simulink model "recordEEGExpe3"  (R2019a)
settings: Solver=VariableStepAuto  StartTime=0.0  StopTime=1000  RelTol=1e-3
undefined symbols (not defined in the file or in its folder): daq
libraries: dsparch4 x3, daqlib x1, dspnetwork x1
settings Model: Creator=Kusunoki  LastModifiedBy=Owner

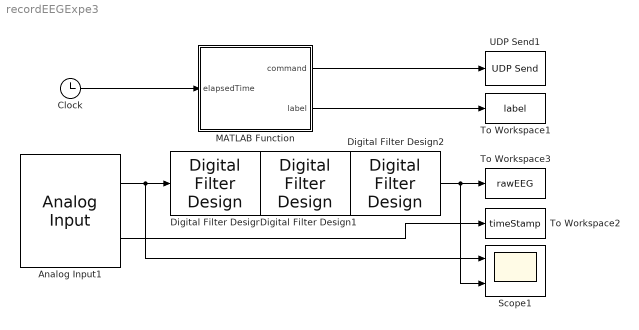
== system recordEEGExpe3 ==
  Analog Input1 : daqlib/Analog Input  DeviceMenu=ni Dev1 (USB-6000)  Device=ni Dev1 (USB-6000)  ObjConstructor=daq.createSession('ni')  NChannelsSelected=8  Channels=1$ai0$$Dev1$1$1$1$1$#1$ai1$$Dev1$1$1$1$1$#1$ai2$$Dev1$1$1$1$1$#1$ai3$$Dev1$1$1$1$1$#1$ai4$$Dev1$1$1$1$1$#1$ai5$$Dev1$1$1$1$1$#1$ai6$$Dev1$1$1$1$1$#1$ai7$$Dev1$1$1$1$1$#  NPorts=1 for all channels  SampleRate=1000  ActualRate=1000  ScansPerTrigger=200  OutputTimestamp=on  AcqMode=0  NumFrameBuffer=100  OutputTriggertime=off
      settings: SourceProductName=Data Acquisition Toolbox  SourceProductBaseCode=DA
  Clock : Clock
  Digital Filter Design : dsparch4/Digital Filter Design  mwdsp_browser_bugfix_var=off
  Digital Filter Design1 : dsparch4/Digital Filter Design  mwdsp_browser_bugfix_var=off
  Digital Filter Design2 : dsparch4/Digital Filter Design  mwdsp_browser_bugfix_var=off
  MATLAB Function : MATLAB Function  TreatAsAtomicUnit=on
  Scope1 : Scope  NumInputPorts=2
  To Workspace1 : ToWorkspace  VariableName=label  SampleTime=(1/1000) * 200
      settings: Save2DSignal=2-D array (concatenate along first dimension)
  To Workspace2 : ToWorkspace  VariableName=timeStamp  SampleTime=-1
      settings: Save2DSignal=2-D array (concatenate along first dimension)
  To Workspace3 : ToWorkspace  VariableName=rawEEG  SampleTime=-1
      settings: Save2DSignal=2-D array (concatenate along first dimension)
  UDP Send1 : dspnetwork/UDP Send  remoteURL='127.0.0.1'  remotePort=25000  localURL='0.0.0.0'  localPortSource=Automatically determine  localPort=-1  sampletime=-1  blockPlatform=[]  separateLengthPort=0
      settings: SourceProductName=Simulink
  wires:
  MATLAB Function/1(command) -> UDP Send1/1
  Analog Input1/2 -> To Workspace2/1
  MATLAB Function/2(label) -> To Workspace1/1
  Analog Input1/1 -> Scope1/1, Digital Filter Design/1
  Digital Filter Design/1 -> Digital Filter Design1/1
  Digital Filter Design1/1 -> Digital Filter Design2/1
  Digital Filter Design2/1 -> Scope1/2, To Workspace3/1
  Clock/1 -> MATLAB Function/1(elapsedTime)

== matlab function recordEEGExpe3/MATLAB Function ==
  data: elapsedTime input; command output size=1; label output size=[200,1]
function [command, label] = commandGenerator(elapsedTime)
    command = cast(0,'uint32');
    interval = 10;%[s]
    if elapsedTime <= (interval * 1)
        command = cast(0,'uint32');;
        
    elseif elapsedTime <= (interval * 2)
        command = cast(303,'uint32');
        
    elseif elapsedTime <= (interval * 3)
        command = cast(300,'uint32');
        
    elseif elapsedTime <= (interval * 4)
        command = cast(301,'uint32');
        
    elseif elapsedTime <= (interval * 5)
        command = cast(0,'uint32');
        
    elseif elapsedTime <= (interval * 6)
        command = cast(302,'uint32');
        
    else 
        %reset to next pattern
        command = cast(0,'uint32');
    end
	
    label = reshape(ones(200,1) * cast(command, 'double'),[200,1]);
end
